simulink model "IO424_LVDT_signal_gen"  (R2024b)
settings: Solver=FixedStepDiscrete  StartTime=0.0  StopTime=0.3  FixedStep=1e-6  RelTol=1e-3
settings Model: Creator=aleandro.vegni  LastModifiedBy=nathan.gyger

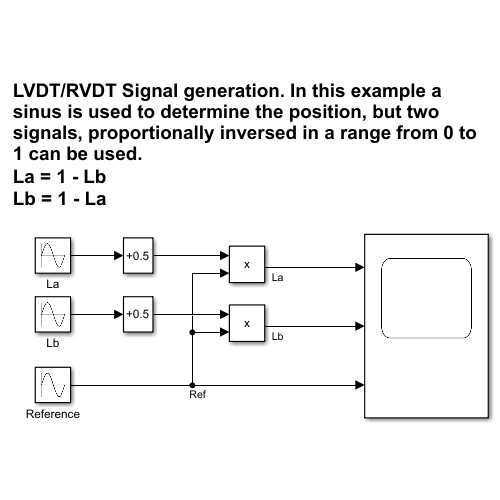
[thumbnail: Simulink's stored preview of the top-level diagram]
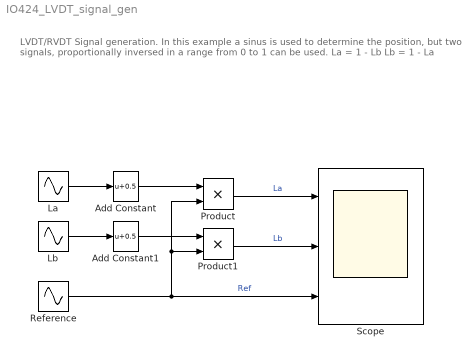
== system IO424_LVDT_signal_gen ==
  note: LVDT/RVDT Signal generation. In this example a sinus is used to determine the position, but two signals, proportionally inversed in a range from 0 to 1 can be used.
      | La = 1 - Lb
      | Lb = 1 - La
  Add Constant : Bias  Bias=0.5  SaturateOnIntegerOverflow=off
  Add Constant1 : Bias  Bias=0.5  SaturateOnIntegerOverflow=off
  La : Sin  Amplitude=0.5  Frequency=2*pi*10  SampleTime=0
  Lb : Sin  Amplitude=0.5  Frequency=2*pi*10  Phase=pi  SampleTime=0
  Product : Product
  Product1 : Product
  Reference : Sin  Amplitude=4*sqrt(2)  Frequency=2*pi*1e3  SampleTime=0
  Scope : Scope  NumInputPorts=3
  wires:
  La/1 -> Add Constant/1
  Reference/1 -> Scope/3, Product/2, Product1/2  "Ref"
  Lb/1 -> Add Constant1/1
  Add Constant1/1 -> Product1/1
  Add Constant/1 -> Product/1
  Product/1 -> Scope/1  "La"
  Product1/1 -> Scope/2  "Lb"
